simulink model "hw2_q2"  (R2020a)
settings: Solver=VariableStepAuto  StartTime=0.0  StopTime=6/100  RelTol=1e-3
libraries: powerlib x10, powerlib_meascontrol x3
settings Model: Creator=tahsi  LastModifiedBy=tahsi
settings DebuggingCC: UnconnectedInputMsg=none  UnconnectedOutputMsg=none  UnconnectedLineMsg=none
settings ModelReferenceCC: EnableRefExpFcnMdlSchedulingChecks=off
settings RTWCC: Description=Generic Real-Time Target

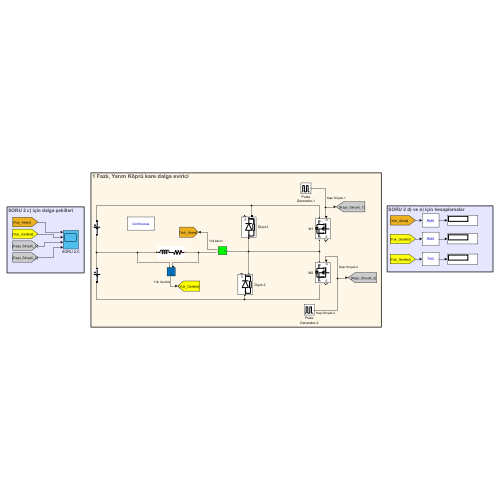
[thumbnail: Simulink's stored preview of the top-level diagram]
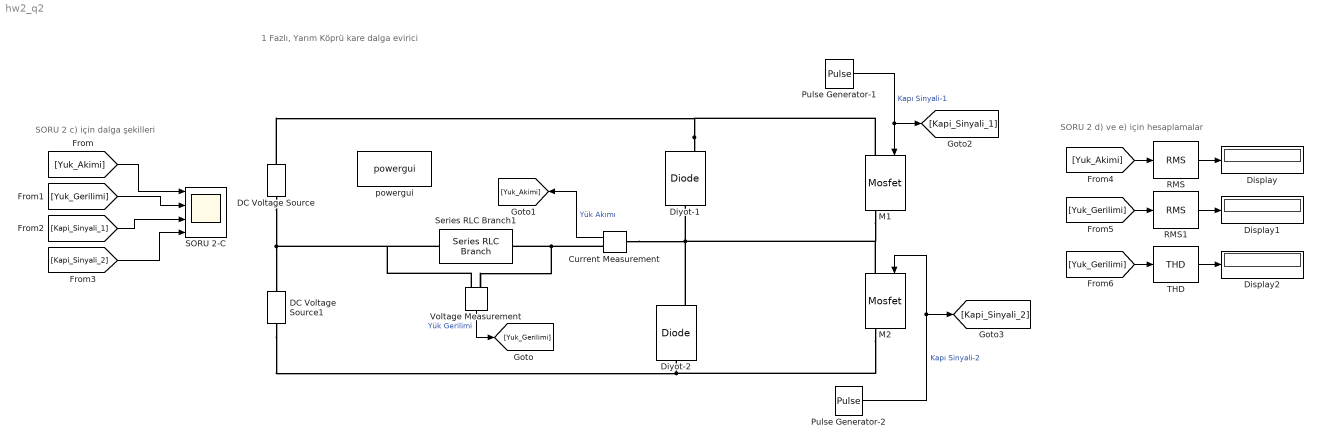
== system hw2_q2 ==
  note: 1 Fazlı, Yarım Köprü kare dalga evirici
  note: SORU 2 d) ve e) için hesaplamalar
  note: SORU 2 c) için dalga şekilleri
  Current Measurement : powerlib/Measurements/Current Measurement  PhasorSimulation=off  OutputType=Complex  PSBequivalent=0
  DC Voltage Source : powerlib/Electrical Sources/DC Voltage Source  Amplitude=25  Measurements=None
  DC Voltage Source1 : powerlib/Electrical Sources/DC Voltage Source  Amplitude=25  Measurements=None
  Display : Display
  Display1 : Display
  Display2 : Display
  Diyot-1 : powerlib/Power Electronics/Diode  Ron=0.001  Lon=0  Vf=0.8  IC=0  UseSnubber=0  Rs=500  Cs=250e-9  Measurements=on
  Diyot-2 : powerlib/Power Electronics/Diode  Ron=0.001  Lon=0  Vf=0.8  IC=0  UseSnubber=0  Rs=500  Cs=250e-9  Measurements=on
  M1 : powerlib/Power Electronics/Mosfet  Ron=0.1  Lon=0  Rd=0.01  Vfd=0  IC=0  Rs=1e5  Cs=inf  Measurements=on
  M2 : powerlib/Power Electronics/Mosfet  Ron=0.1  Lon=0  Rd=0.01  Vfd=0  IC=0  Rs=1e5  Cs=inf  Measurements=on
  Pulse Generator-1 : DiscretePulseGenerator  PulseType=Time based  Period=1/50  PulseWidth=50
  Pulse Generator-2 : DiscretePulseGenerator  PulseType=Time based  Period=1/50  PulseWidth=50  PhaseDelay=1/100
  RMS : powerlib_meascontrol/Measurements/RMS  TrueRMS=on  Freq=50  RMSInit=120  Ts=0
  RMS1 : powerlib_meascontrol/Measurements/RMS  TrueRMS=on  Freq=50  RMSInit=120  Ts=0
  SORU 2-C : Scope  NumInputPorts=4
  Series RLC Branch1 : powerlib/Elements/Series RLC Branch  LConnTagsString=__new0  RConnTagsString=__new0  BranchType=RL  Resistance=10  Inductance=20e-3  SetiL0=off  InitialCurrent=0  Capacitance=1e-6  Setx0=off  InitialVoltage=0  Measurements=None
  THD : powerlib_meascontrol/Measurements/THD  Freq=50  Ts=0
  Voltage Measurement : powerlib/Measurements/Voltage Measurement  PhasorSimulation=off  OutputType=Complex  PSBequivalent=0
  powergui : powerlib/powergui  Priority=1  SimulationMode=Continuous  SampleTime=50e-6  frequency=60  Iterations=50  frequencyindice=0  Pbase=100e6  ErrMax=1e-4  UnitsV=kV  UnitsW=MW  buscounter=0  FunctionMessages=off  echomessages=off  EnableUseOfTLC=off  CurrentSourceSwitches=off  DisableSnubberDevices=off  DisableRonSwitches=off  DisableVfSwitches=off  DisplayEquations=off  AutomaticDiscreteSolvers=off  SolverType=Tustin/Backward Euler (TBE)  Interpol=off  ExternalGateDelay=off  methode=off  Ts=100  x0status=blocks  SPID=on  SwTol=0  HookPort=off  NonlinearTolerance=1e-4  nMaxIteration=100  ContinueOnMaxIteration=off  RestoreLinks=warning  ResistiveCurrentMeasurement=off  Frange=[0:2:500]  Ylog=off  Xlog=on  ShowGrid=off  save=off  variable=ZData  structure=0  ZoomFFT=off  StartTime=0.0  cycles=1  DisplayStyle=1  fundamental=60  FreqAxis=off  MaxFrequency=1000  frequencyindicesteady=1  RmsSteady=1  display=off
  wires:
  Pulse Generator-1/1 -> M1/1, [Kapi_Sinyali_1]  "Kapı Sinyali-1"
  Pulse Generator-2/1 -> [Kapi_Sinyali_2], M2/1  "Kapı Sinyali-2"
  Voltage Measurement/1 -> [Yuk_Gerilimi]  "Yük Gerilimi"
  Current Measurement/1 -> [Yuk_Akimi]  "Yük Akımı"
  [Yuk_Akimi] -> SORU 2-C/1
  [Yuk_Gerilimi] -> SORU 2-C/2
  [Kapi_Sinyali_1] -> SORU 2-C/3
  [Kapi_Sinyali_2] -> SORU 2-C/4
  [Yuk_Akimi] -> RMS/1
  RMS/1 -> Display/1
  [Yuk_Gerilimi] -> RMS1/1
  RMS1/1 -> Display1/1
  [Yuk_Gerilimi] -> THD/1
  THD/1 -> Display2/1
  connections:
  Diyot-2/RConn1 -- Current Measurement/LConn1 -- M2/LConn1 -- M1/RConn1 -- Diyot-1/LConn1
  DC Voltage Source/LConn1 -- Series RLC Branch1/RConn1 -- Voltage Measurement/LConn2 -- DC Voltage Source1/RConn1
  Diyot-1/RConn1 -- DC Voltage Source/RConn1 -- M1/LConn1
  DC Voltage Source1/LConn1 -- M2/RConn1 -- Diyot-2/LConn1
  Voltage Measurement/LConn1 -- Series RLC Branch1/LConn1 -- Current Measurement/RConn1
